simulink model "lab1_model"  (Simulink 7.6)
settings: Solver=ode45  StartTime=0.0  StopTime=20  RelTol=1e-3
values from neighbouring files (symbols this model uses):
  cpw = 4190    [skrypt.m]    (also in symulacja_dyn.m = cpw_; testerka.m)
  Cvg = cpw*row*Vg    (= 410620)    [skrypt.m]    (also in symulacja_dyn.m = cpw*row*Vg)
  Cvw = cpp*rop*Vp*3    (= 268758)    [skrypt.m]    (also in symulacja_dyn.m = cpp*rop*Vp*3)
  dFg = 0    [skrypt.m]    (also in symulacja_dyn.m = dFg_; testerka.m)
  dQt = 0    [skrypt.m]    (also in symulacja_dyn.m = dQt_; testerka.m)
  dt = 5    [skrypt.m]    (also in symulacja_dyn.m)
  dTgz = 0    [skrypt.m]    (also in symulacja_dyn.m = dTgz_; testerka.m)
  dTzew = 0    [skrypt.m]    (also in symulacja_dyn.m = dTzew_; testerka.m = -20)
  Fg_0 = Fg_n    (= 0.000243534167844)    [skrypt.m]    (also in symulacja_dyn.m = Fg_n; testerka.m = Fg_0 * 2)
  kg = Q_n/(Tgsr_n-Twew_n)    (= 400)    [skrypt.m]    (also in symulacja_dyn.m = Q_n/(Tgsr_n-Twew_n))
  kw = (Q_n-Qt_0)/(Twew_n-Tzew_n)    (= 500)    [skrypt.m]    (also in symulacja_dyn.m = (Q_n-Qt_0)/(Twew_n-Tzew_n))
  Qt_0 = 0    [skrypt.m]    (also in symulacja_dyn.m)
  row = 980    [skrypt.m]    (also in symulacja_dyn.m = row_; testerka.m)
  Tgsr_0 = Tgsr_n    (= 70)    [skrypt.m]    (also in symulacja_dyn.m = Tgsr_n)
  Tgz_0 = Tgz_n    (= 90)    [skrypt.m]    (also in symulacja_dyn.m = Tgz_n; testerka.m)
  Twew_0 = Twew_n    (= 20)    [skrypt.m]    (also in symulacja_dyn.m = Twew_n)
  Tzew_0 = Tzew_n    (= -20)    [skrypt.m]    (also in symulacja_dyn.m = Tzew_n; testerka.m = Tzew_0 - 10)
settings Model: Creator=LAB320-1537-User  LastModifiedBy=qrczak
settings DebuggingCC: FcnCallInpInsideContextMsg=Enable All
settings GRTTargetCC: CombineOutputUpdateFcns=on

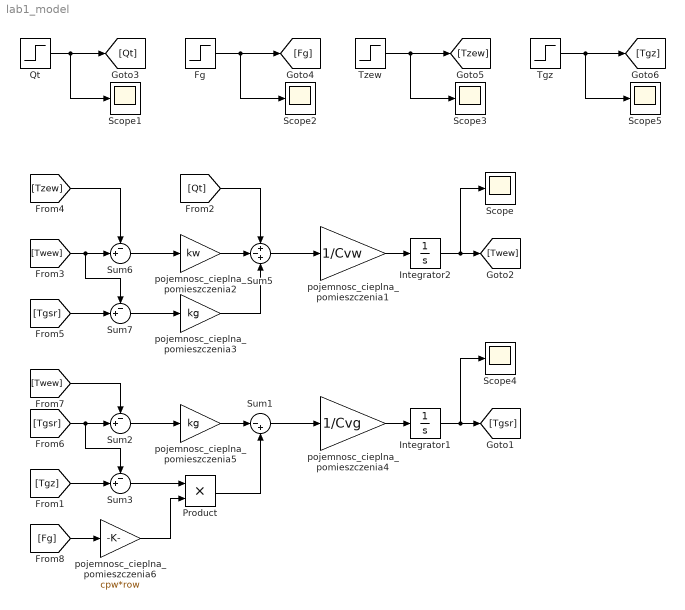
== system lab1_model ==
  Fg : Step  Time=dt  Before=Fg_0  After=Fg_0+dFg  SampleTime=0
  Integrator1 : Integrator  InitialCondition=Tgsr_0
  Integrator2 : Integrator  InitialCondition=Twew_0
  Product : Product  RndMeth=Zero
  Qt : Step  Time=dt  Before=Qt_0  After=Qt_0+dQt  SampleTime=0
  Scope{,1..5} (6 alike) : Scope
      Scope settings: SaveName=ScopeData2
      Scope1 settings: SaveName=ScopeData3
      Scope3 settings: SaveName=ScopeData5
      Scope5 settings: SaveName=ScopeData4
  Sum1 : Sum  Inputs=|-+
  Sum{2..3,6..7} (4 alike) : Sum  Inputs=-+|
  Sum5 : Sum  Inputs=+-+
  Tgz : Step  Time=dt  Before=Tgz_0  After=Tgz_0+dTgz  SampleTime=0
  Tzew : Step  Time=dt  Before=Tzew_0  After=Tzew_0+dTzew  SampleTime=0
  pojemnosc_cieplna_pomieszczenia1 : Gain  Gain=1/Cvw
  pojemnosc_cieplna_pomieszczenia2 : Gain  Gain=kw
  pojemnosc_cieplna_pomieszczenia3 : Gain  Gain=kg
  pojemnosc_cieplna_pomieszczenia4 : Gain  Gain=1/Cvg
  pojemnosc_cieplna_pomieszczenia5 : Gain  Gain=kg
  pojemnosc_cieplna_pomieszczenia6 : Gain  Gain=cpw*row
  wires:
  pojemnosc_cieplna_pomieszczenia1/1 -> Integrator2/1
  Integrator2/1 -> [Twew], Scope/1
  Qt/1 -> [Qt], Scope1/1
  Tzew/1 -> Scope3/1, [Tzew]
  Sum5/1 -> pojemnosc_cieplna_pomieszczenia1/1
  [Qt] -> Sum5/1
  pojemnosc_cieplna_pomieszczenia2/1 -> Sum5/2
  pojemnosc_cieplna_pomieszczenia3/1 -> Sum5/3
  Sum6/1 -> pojemnosc_cieplna_pomieszczenia2/1
  [Twew] -> Sum6/2, Sum7/1
  [Tzew] -> Sum6/1
  [Tgsr] -> Sum7/2
  Sum7/1 -> pojemnosc_cieplna_pomieszczenia3/1
  pojemnosc_cieplna_pomieszczenia4/1 -> Integrator1/1
  Integrator1/1 -> [Tgsr], Scope4/1
  Sum1/1 -> pojemnosc_cieplna_pomieszczenia4/1
  Sum2/1 -> pojemnosc_cieplna_pomieszczenia5/1
  [Tgsr] -> Sum2/2, Sum3/1
  [Twew] -> Sum2/1
  pojemnosc_cieplna_pomieszczenia5/1 -> Sum1/1
  [Tgz] -> Sum3/2
  [Fg] -> pojemnosc_cieplna_pomieszczenia6/1
  pojemnosc_cieplna_pomieszczenia6/1 -> Product/2
  Sum3/1 -> Product/1
  Product/1 -> Sum1/2
  Fg/1 -> Scope2/1, [Fg]
  Tgz/1 -> Scope5/1, [Tgz]
